simulink model "rccg_digitalTwin_scenario1"  (R2024a)
settings: Solver=VariableStepAuto  StartTime=0.0  StopTime=5  RelTol=1e-3
libraries: spsThreePhaseVIMeasurementLib x11, spsThreePhaseBreakerLib x9, spsThreePhaseDynamicLoadLib x7, spsSynchronousMachinepuStandardLib x2, spsThreePhaseParallelRLCLoadLib x2, spsThreePhaseTransformerTwoWindingsLib x1, spsExcitationSystemLib x1, spsHydraulicTurbineandGovernorLib x1, sps_lib x1
settings Model: Creator=dogba  LastModifiedBy=dogba

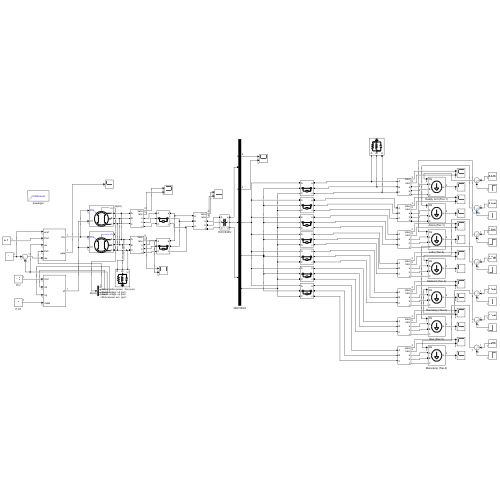
[thumbnail: Simulink's stored preview of the top-level diagram]
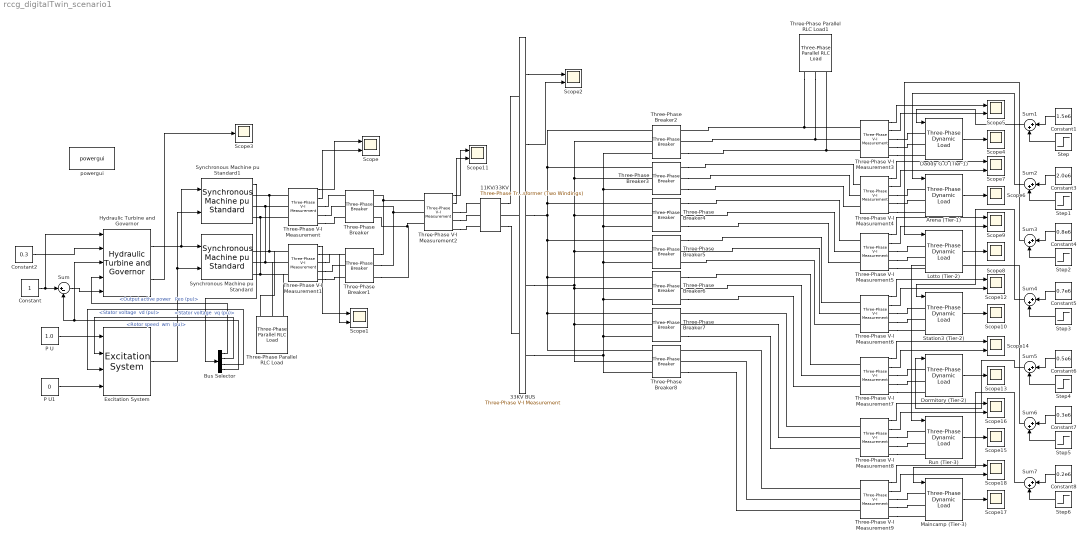
== system rccg_digitalTwin_scenario1 ==
  11KV/33KV : spsThreePhaseTransformerTwoWindingsLib/Three-Phase Transformer (Two Windings)  Winding1Connection=Yg  Winding2Connection=Yg  CoreType=Three single-phase transformers  SetSaturation=off  Hysteresis=off  DataFile='hysteresis'  SetInitialFlux=off  Measurements=None  UNITS=pu  NominalPower=[ 10e6 , 60 ]  Winding1=[ 11e3 , 0.002 , 0.08 ]  Winding2=[ 33e3 , 0.002 , 0.08 ]  Rm=500  Lm=500  L0=0.5  Saturation=[ 0,0 ; 0.0024,1.2 ; 1.0,1.52 ]  InitialFluxes=[ 0.8 , -0.8 , 0.7 ]  BreakLoop=off  DiscreteSolver=Trapezoidal iterative  DataType=off  TransfoNumber=1
  33KV BUS : spsThreePhaseVIMeasurementLib/Three-Phase V-I Measurement  VoltageMeasurement=phase-to-ground  SetLabelV=off  LabelV=Vabc  Vpu=off  VpuLL=off  CurrentMeasurement=yes  SetLabelI=off  LabelI=Iabc  Ipu=off  Pbase=100e6  Vbase=500e3  OutputType=Complex  PhasorSimulation=off  PSBequivalent=0
  Arena (Tier-1) : spsThreePhaseDynamicLoadLib/Three-Phase Dynamic Load  NominalVoltage=[ 415 50 ]  ActiveReactivePowers=[1.5e6 0.4e6]  PositiveSequence=[0.994 -11.8]  ExternalControl=on  NpNq=[1.3 2]  TimeConstants="[0  0  0  0]"  MinimumVoltage=0.7  Tfilter=1e-4  LoadFlowParameters=[4,0,0,0,0]
      settings: LibrarySourceBlock=|
      | sps_lib/Passives/Three-Phase
      | Dynamic Load
  Bus Selector : BusSelector  OutputSignals="Output active power   Peo (pu),dq0 components.Stator voltage  vd (pu),dq0 components.Stator voltage  vq (pu),Mechanical.Rotor speed  wm  (pu)"
  Constant : Constant
  Constant1 : Constant  Value=1.5e6
  Constant2 : Constant  Value=0.3
  Constant3 : Constant  Value=2.0e6
  Constant4 : Constant  Value=0.8e6
  Constant5 : Constant  Value=0.7e6
  Constant6 : Constant  Value=0.5e6
  Constant7 : Constant  Value=0.3e6
  Constant8 : Constant  Value=0.2e6
  Daddy G.O (Tier-1) : spsThreePhaseDynamicLoadLib/Three-Phase Dynamic Load  NominalVoltage=[ 415 50 ]  ActiveReactivePowers=[1.5e6 0.4e6]  PositiveSequence=[0.994 -11.8]  ExternalControl=on  NpNq=[1.3 2]  TimeConstants="[0  0  0  0]"  MinimumVoltage=0.7  Tfilter=1e-4  LoadFlowParameters=[4,0,0,0,0]
      settings: LibrarySourceBlock=|
      | sps_lib/Passives/Three-Phase
      | Dynamic Load
  Dormitory (Tier-2) : spsThreePhaseDynamicLoadLib/Three-Phase Dynamic Load  NominalVoltage=[ 415 50 ]  ActiveReactivePowers=[1.5e6 0.4e6]  PositiveSequence=[0.994 -11.8]  ExternalControl=on  NpNq=[1.3 2]  TimeConstants="[0  0  0  0]"  MinimumVoltage=0.7  Tfilter=1e-4  LoadFlowParameters=[4,0,0,0,0]
      settings: LibrarySourceBlock=|
      | sps_lib/Passives/Three-Phase
      | Dynamic Load
  Excitation System : spsExcitationSystemLib/Excitation System  tr=20e-3  reg=[ 300, 0.001 ]  exc=[ 1, 0 ]  tgr=[ 0, 0 ]  damp=[ 0.001, 0.1 ]  sat=[ 0, 0 ]  lim=[ -11.5, 11.5, 0 ]  v0="[1.0  1.28]"
      settings: LibrarySourceBlock=sps_lib/Electrical Machines/Synchronous Machine Control/Excitation System
  Hydraulic Turbine and Governor : spsHydraulicTurbineandGovernorLib/Hydraulic Turbine and Governor  sm="[ 10/3  0.07 ]"  gate="[  0.01  0.97518  -0.1  0.1 ]"  reg="[  0.05  1.163  0.105  0  0.01  ]"  hyd="[  0  2.67  ]"  dref=0  po=0.7516
      settings: LibrarySourceBlock=|
      | sps_lib/Electrical Machines/Synchronous Machine Control/Hydraulic Turbine
      | and Governor
  Lotto (Tier-2) : spsThreePhaseDynamicLoadLib/Three-Phase Dynamic Load  NominalVoltage=[ 415 50 ]  ActiveReactivePowers=[1.5e6 0.4e6]  PositiveSequence=[0.994 -11.8]  ExternalControl=on  NpNq=[1.3 2]  TimeConstants="[0  0  0  0]"  MinimumVoltage=0.7  Tfilter=1e-4  LoadFlowParameters=[4,0,0,0,0]
      settings: LibrarySourceBlock=|
      | sps_lib/Passives/Three-Phase
      | Dynamic Load
  Maincamp (Tier-3) : spsThreePhaseDynamicLoadLib/Three-Phase Dynamic Load  NominalVoltage=[ 415 50 ]  ActiveReactivePowers=[1.5e6 0.4e6]  PositiveSequence=[0.994 -11.8]  ExternalControl=on  NpNq=[1.3 2]  TimeConstants="[0  0  0  0]"  MinimumVoltage=0.7  Tfilter=1e-4  LoadFlowParameters=[4,0,0,0,0]
      settings: LibrarySourceBlock=|
      | sps_lib/Passives/Three-Phase
      | Dynamic Load
  P U : Constant  Value=1.0
  P U1 : Constant  Value=0
  Run (Tier-3) : spsThreePhaseDynamicLoadLib/Three-Phase Dynamic Load  NominalVoltage=[ 415 50 ]  ActiveReactivePowers=[1.5e6 0.4e6]  PositiveSequence=[0.994 -11.8]  ExternalControl=on  NpNq=[1.3 2]  TimeConstants="[0  0  0  0]"  MinimumVoltage=0.7  Tfilter=1e-4  LoadFlowParameters=[4,0,0,0,0]
      settings: LibrarySourceBlock=|
      | sps_lib/Passives/Three-Phase
      | Dynamic Load
  Scope{,1..2,5,7,9,11..12,14,16,18} (11 alike) : Scope  NumInputPorts=2
  Scope{3..4,6,8,10,13,15,17} (8 alike) : Scope
  "Station3 (Tier-2) " : spsThreePhaseDynamicLoadLib/Three-Phase Dynamic Load  NominalVoltage=[ 415 50 ]  ActiveReactivePowers=[1.5e6 0.4e6]  PositiveSequence=[0.994 -11.8]  ExternalControl=on  NpNq=[1.3 2]  TimeConstants="[0  0  0  0]"  MinimumVoltage=0.7  Tfilter=1e-4  LoadFlowParameters=[4,0,0,0,0]
      settings: LibrarySourceBlock=|
      | sps_lib/Passives/Three-Phase
      | Dynamic Load
  Step : Step  Time=2.5  After=0.78e6  SampleTime=0
  Step1 : Step  Time=2.5  After=1.6e6  SampleTime=0
  Step{2..6} (5 alike) : Step  Time=2.5  After=0  SampleTime=0
  Sum : Sum  Inputs=|+-
  Sum{1..7} (7 alike) : Sum  Inputs=|++
  Synchronous Machine pu Standard : spsSynchronousMachinepuStandardLib/Synchronous Machine pu Standard  PresetModel=No  MechanicalLoad=Mechanical power Pm  ShowDetailedParameters=on  RotorType=Salient-pole  Units=per unit standard parameters  MeasurementBus=off  NominalParameters=[5e6 11e3 50]  Reactances1=[ 1.81, 0.3, 0.23, 1.76, 0.65, 0.25, 0.15 ]  Reactances2=[2.24 0.17 0.12 1.02 0.13 0.08]  dAxisTimeConstants=Short-circuit  qAxisTimeConstants=Short-circuit  TimeConstants1="[ 4.4849  0.0681  0.1  ]"  TimeConstants2=[ 8.0, 0.03, 1.0, 0.07 ]  TimeConstants3="[  4.49  0.0681  0.0513  ]"  TimeConstants4=[ 8.0, 0.03, 0.3371, 0.0295 ]  TimeConstants5=[ 1.01, 0.053, 0.1 ]  TimeConstants6=[ 1.3201, 0.023, 1.0, 0.07 ]  TimeConstants7=[0.012 0.003 0.003]  TimeConstants8=[ 1.3201, 0.0231, 0.3371, 0.0295 ]  StatorResistance=0.037875  Mechanical=[0.1028 0.02056 2]  PolePairs=20  InitialConditions="[ 0  0  0  0  0  0  0  0  1 ]"  SetSaturation=on  Saturation=[0.6404,0.7127,0.8441,0.9214,0.9956,1.082,1.19,1.316,1.457;0.7,0.7698,0.8872,0.9466,0.9969,1.046,1.1,1.151,1.201]  LoadFlowParameters=[1,0,0,0,0]  TsPowergui=0  TsBlock=-1  IterativeModel=Trapezoidal non iterative  IterativeDiscreteModel=Trapezoidal non iterative  BusType=PV  Pref=0  Qref=0  Qmin=-inf  Qmax=inf  PLF=0  QLF=0
  Synchronous Machine pu Standard1 : spsSynchronousMachinepuStandardLib/Synchronous Machine pu Standard  PresetModel=No  MechanicalLoad=Mechanical power Pm  ShowDetailedParameters=on  RotorType=Salient-pole  Units=per unit standard parameters  MeasurementBus=off  NominalParameters=[5e6 11e3 50]  Reactances1=[ 1.81, 0.3, 0.23, 1.76, 0.65, 0.25, 0.15 ]  Reactances2=[2.24 0.17 0.12 1.02 0.13 0.08]  dAxisTimeConstants=Short-circuit  qAxisTimeConstants=Short-circuit  TimeConstants1="[ 4.4849  0.0681  0.1  ]"  TimeConstants2=[ 8.0, 0.03, 1.0, 0.07 ]  TimeConstants3="[  4.49  0.0681  0.0513  ]"  TimeConstants4=[ 8.0, 0.03, 0.3371, 0.0295 ]  TimeConstants5=[ 1.01, 0.053, 0.1 ]  TimeConstants6=[ 1.3201, 0.023, 1.0, 0.07 ]  TimeConstants7=[0.012 0.003 0.003]  TimeConstants8=[ 1.3201, 0.0231, 0.3371, 0.0295 ]  StatorResistance=0.037875  Mechanical=[0.1028 0.02056 2]  PolePairs=20  InitialConditions="[ 0  0  0  0  0  0  0  0  1 ]"  SetSaturation=on  Saturation=[0.6404,0.7127,0.8441,0.9214,0.9956,1.082,1.19,1.316,1.457;0.7,0.7698,0.8872,0.9466,0.9969,1.046,1.1,1.151,1.201]  LoadFlowParameters=[1,0,0,0,0]  TsPowergui=0  TsBlock=-1  IterativeModel=Trapezoidal non iterative  IterativeDiscreteModel=Trapezoidal non iterative  BusType=PV  Pref=0  Qref=0  Qmin=-inf  Qmax=inf  PLF=0  QLF=0
  Three-Phase Parallel RLC Load : spsThreePhaseParallelRLCLoadLib/Three-Phase Parallel RLC Load  LConnTagsString=A|B|C  Configuration=Y (grounded)  NominalVoltage=1000  Vabc=[1e3 1e3 1e3]  Vabcp=[1e3 1e3 1e3]  NominalFrequency=60  UnbalancedPower=off  ActivePower=10e3  InductivePower=100  CapacitivePower=100  Pabc=[10e3 9e3 11e3]  QLabc=[100 90 110]  QCabc=[100 90 110]  Pabcp=[10e3 9e3 11e3]  QLabcp=[100 90 110]  QCabcp=[100 90 110]  Measurements=None  LoadType=constant Z
  Three-Phase Parallel RLC Load1 : spsThreePhaseParallelRLCLoadLib/Three-Phase Parallel RLC Load  LConnTagsString=A|B|C  Configuration=Y (grounded)  NominalVoltage=1000  Vabc=[1e3 1e3 1e3]  Vabcp=[1e3 1e3 1e3]  NominalFrequency=60  UnbalancedPower=off  ActivePower=10e3  InductivePower=100  CapacitivePower=100  Pabc=[10e3 9e3 11e3]  QLabc=[100 90 110]  QCabc=[100 90 110]  Pabcp=[10e3 9e3 11e3]  QLabcp=[100 90 110]  QCabcp=[100 90 110]  Measurements=None  LoadType=constant Z
  Three-Phase V-I Measurement{,1..9} (10 alike) : spsThreePhaseVIMeasurementLib/Three-Phase V-I Measurement  VoltageMeasurement=phase-to-ground  SetLabelV=off  LabelV=Vabc  Vpu=off  VpuLL=off  CurrentMeasurement=yes  SetLabelI=off  LabelI=Iabc  Ipu=off  Pbase=100e6  Vbase=500e3  OutputType=Complex  PhasorSimulation=off  PSBequivalent=0
  Three-Phase Breaker{,1..8} (9 alike) : spsThreePhaseBreakerLib/Three-Phase Breaker  InitialState=closed  SwitchA=on  SwitchB=on  SwitchC=on  SwitchTimes="[1/60  5/60]"  External=off  BreakerResistance=0.01  SnubberResistance=1e6  SnubberCapacitance=inf  Measurements=None
  powergui : sps_lib/powergui  Priority=1  SimulationMode=Continuous  SampleTime=50e-6  frequency=60  Iterations=50  frequencyindice=50  Pbase=100e6  ErrMax=1e-4  UnitsV=kV  UnitsW=MW  buscounter=0  FunctionMessages=off  echomessages=off  EnableUseOfTLC=off  CurrentSourceSwitches=off  DisableSnubberDevices=off  DisableRonSwitches=off  DisableVfSwitches=off  DisplayEquations=off  AutomaticDiscreteSolvers=off  SolverType=Tustin/Backward Euler (TBE)  Interpol=off  ExternalGateDelay=off  methode=off  Ts=100  x0status=blocks  SPID=on  SwTol=0  HookPort=off  NonlinearTolerance=1e-4  nMaxIteration=100  ContinueOnMaxIteration=off  RestoreLinks=warning  ResistiveCurrentMeasurement=off  Frange=[0:2:500]  Ylog=off  Xlog=on  ShowGrid=off  save=off  variable=ZData  structure=0  ZoomFFT=off  StartTime=0.0  cycles=1  DisplayStyle=1  fundamental=60  FreqAxis=off  MaxFrequency=1000  frequencyindicesteady=1  RmsSteady=1  display=off
  wires:
  Excitation System/1 -> Synchronous Machine pu Standard1/2, Synchronous Machine pu Standard/2
  Hydraulic Turbine and Governor/1 -> Synchronous Machine pu Standard1/1, Synchronous Machine pu Standard/1
  P U/1 -> Excitation System/1
  P U1/1 -> Excitation System/4
  Three-Phase V-I Measurement/1 -> Scope/1
  Three-Phase V-I Measurement/2 -> Scope/2
  Three-Phase V-I Measurement1/1 -> Scope1/1
  Three-Phase V-I Measurement1/2 -> Scope1/2
  Synchronous Machine pu Standard1/1 -> Bus Selector/1
  Bus Selector/1 -> Hydraulic Turbine and Governor/4  "<Output active power   Peo (pu)>"
  Bus Selector/2 -> Excitation System/2  "<Stator voltage  vd (pu)>"
  Bus Selector/3 -> Excitation System/3  "<Stator voltage  vq (pu)>"
  Bus Selector/4 -> Sum/2, Hydraulic Turbine and Governor/3  "<Rotor speed  wm  (pu)>"
  Constant/1 -> Hydraulic Turbine and Governor/1, Sum/1
  Sum/1 -> Hydraulic Turbine and Governor/5
  Constant2/1 -> Hydraulic Turbine and Governor/2
  33KV BUS/1 -> Scope2/1
  33KV BUS/2 -> Scope2/2
  Hydraulic Turbine and Governor/2 -> Scope3/1
  Three-Phase V-I Measurement2/1 -> Scope11/1
  Three-Phase V-I Measurement2/2 -> Scope11/2
  Daddy G.O (Tier-1)/1 -> Scope4/1
  Three-Phase V-I Measurement3/1 -> Scope5/1
  Three-Phase V-I Measurement3/2 -> Scope5/2
  Three-Phase V-I Measurement4/2 -> Scope7/2
  Three-Phase V-I Measurement4/1 -> Scope7/1
  Arena (Tier-1)/1 -> Scope6/1
  Lotto (Tier-2)/1 -> Scope8/1
  Three-Phase V-I Measurement5/1 -> Scope9/1
  Three-Phase V-I Measurement5/2 -> Scope9/2
  Three-Phase V-I Measurement6/2 -> Scope12/2
  Three-Phase V-I Measurement6/1 -> Scope12/1
  "Station3 (Tier-2) "/1 -> Scope10/1
  Dormitory (Tier-2)/1 -> Scope13/1
  Three-Phase V-I Measurement7/1 -> Scope14/1
  Three-Phase V-I Measurement7/2 -> Scope14/2
  Three-Phase V-I Measurement8/2 -> Scope16/2
  Three-Phase V-I Measurement8/1 -> Scope16/1
  Run (Tier-3)/1 -> Scope15/1
  Maincamp (Tier-3)/1 -> Scope17/1
  Three-Phase V-I Measurement9/1 -> Scope18/1
  Three-Phase V-I Measurement9/2 -> Scope18/2
  Constant1/1 -> Sum1/1
  Step/1 -> Sum1/2
  Sum1/1 -> Daddy G.O (Tier-1)/1
  Sum2/1 -> Arena (Tier-1)/1
  Step1/1 -> Sum2/2
  Constant3/1 -> Sum2/1
  Constant5/1 -> Sum4/1
  Step3/1 -> Sum4/2
  Sum4/1 -> "Station3 (Tier-2) "/1
  Sum3/1 -> Lotto (Tier-2)/1
  Step2/1 -> Sum3/2
  Constant4/1 -> Sum3/1
  Constant7/1 -> Sum6/1
  Step5/1 -> Sum6/2
  Sum6/1 -> Run (Tier-3)/1
  Sum7/1 -> Maincamp (Tier-3)/1
  Step6/1 -> Sum7/2
  Constant8/1 -> Sum7/1
  Constant6/1 -> Sum5/1
  Step4/1 -> Sum5/2
  Sum5/1 -> Dormitory (Tier-2)/1
  connections:
  Three-Phase Breaker1/RConn1 -- Three-Phase Breaker/RConn1 -- Three-Phase V-I Measurement2/LConn1
  Three-Phase Breaker1/RConn2 -- Three-Phase Breaker/RConn2 -- Three-Phase V-I Measurement2/LConn2
  Three-Phase Breaker1/RConn3 -- Three-Phase V-I Measurement2/LConn3 -- Three-Phase Breaker/RConn3
  33KV BUS/LConn2 -- 11KV/33KV/RConn2
  11KV/33KV/RConn1 -- 33KV BUS/LConn1
  11KV/33KV/RConn3 -- 33KV BUS/LConn3
  Three-Phase V-I Measurement/LConn1 -- Three-Phase Parallel RLC Load/LConn1 -- Three-Phase V-I Measurement1/LConn1 -- Synchronous Machine pu Standard/RConn1 -- Synchronous Machine pu Standard1/RConn1
  Three-Phase V-I Measurement/LConn2 -- Synchronous Machine pu Standard1/RConn2 -- Three-Phase Parallel RLC Load/LConn2 -- Three-Phase V-I Measurement1/LConn2 -- Synchronous Machine pu Standard/RConn2
  Three-Phase V-I Measurement/LConn3 -- Three-Phase Parallel RLC Load/LConn3 -- Three-Phase V-I Measurement1/LConn3 -- Synchronous Machine pu Standard/RConn3 -- Synchronous Machine pu Standard1/RConn3
  Three-Phase V-I Measurement1/RConn2 -- Three-Phase Breaker1/LConn2
  Three-Phase V-I Measurement1/RConn3 -- Three-Phase Breaker1/LConn3
  Three-Phase V-I Measurement1/RConn1 -- Three-Phase Breaker1/LConn1
  Three-Phase V-I Measurement/RConn3 -- Three-Phase Breaker/LConn3
  Three-Phase V-I Measurement/RConn2 -- Three-Phase Breaker/LConn2
  Three-Phase V-I Measurement/RConn1 -- Three-Phase Breaker/LConn1
  Three-Phase Breaker8/LConn1 -- Three-Phase Breaker7/LConn1 -- Three-Phase Breaker6/LConn1 -- Three-Phase Breaker5/LConn1 -- 33KV BUS/RConn1 -- Three-Phase Breaker4/LConn1 -- Three-Phase Breaker3/LConn1 -- Three-Phase Breaker2/LConn1
  Three-Phase Breaker2/LConn2 -- Three-Phase Breaker3/LConn2 -- Three-Phase Breaker4/LConn2 -- Three-Phase Breaker5/LConn2 -- 33KV BUS/RConn2 -- Three-Phase Breaker6/LConn2 -- Three-Phase Breaker7/LConn2 -- Three-Phase Breaker8/LConn2
  Three-Phase Breaker2/LConn3 -- Three-Phase Breaker3/LConn3 -- Three-Phase Breaker8/LConn3 -- 33KV BUS/RConn3 -- Three-Phase Breaker7/LConn3 -- Three-Phase Breaker6/LConn3 -- Three-Phase Breaker5/LConn3 -- Three-Phase Breaker4/LConn3
  Three-Phase V-I Measurement2/RConn1 -- 11KV/33KV/LConn1
  Three-Phase V-I Measurement2/RConn2 -- 11KV/33KV/LConn2
  Three-Phase V-I Measurement2/RConn3 -- 11KV/33KV/LConn3
  Three-Phase Parallel RLC Load1/LConn1 -- Three-Phase Breaker2/RConn1 -- Three-Phase V-I Measurement3/LConn1
  Three-Phase Parallel RLC Load1/LConn2 -- Three-Phase V-I Measurement3/LConn2 -- Three-Phase Breaker2/RConn2
  Three-Phase Breaker2/RConn3 -- Three-Phase Parallel RLC Load1/LConn3 -- Three-Phase V-I Measurement3/LConn3
  Three-Phase V-I Measurement3/RConn3 -- Daddy G.O (Tier-1)/LConn3
  Three-Phase V-I Measurement3/RConn2 -- Daddy G.O (Tier-1)/LConn2
  Three-Phase V-I Measurement3/RConn1 -- Daddy G.O (Tier-1)/LConn1
  Three-Phase V-I Measurement4/RConn1 -- Arena (Tier-1)/LConn1
  Three-Phase V-I Measurement4/RConn3 -- Arena (Tier-1)/LConn3
  Three-Phase V-I Measurement4/RConn2 -- Arena (Tier-1)/LConn2
  Three-Phase V-I Measurement5/RConn2 -- Lotto (Tier-2)/LConn2
  Three-Phase V-I Measurement5/RConn3 -- Lotto (Tier-2)/LConn3
  Three-Phase V-I Measurement5/RConn1 -- Lotto (Tier-2)/LConn1
  Three-Phase V-I Measurement6/RConn1 -- "Station3 (Tier-2) "/LConn1
  Three-Phase V-I Measurement6/RConn3 -- "Station3 (Tier-2) "/LConn3
  Three-Phase V-I Measurement6/RConn2 -- "Station3 (Tier-2) "/LConn2
  Three-Phase V-I Measurement7/RConn2 -- Dormitory (Tier-2)/LConn2
  Three-Phase V-I Measurement7/RConn3 -- Dormitory (Tier-2)/LConn3
  Three-Phase V-I Measurement7/RConn1 -- Dormitory (Tier-2)/LConn1
  Three-Phase V-I Measurement8/RConn3 -- Run (Tier-3)/LConn3
  Three-Phase V-I Measurement8/RConn2 -- Run (Tier-3)/LConn2
  Three-Phase V-I Measurement8/RConn1 -- Run (Tier-3)/LConn1
  Three-Phase V-I Measurement9/RConn1 -- Maincamp (Tier-3)/LConn1
  Three-Phase V-I Measurement9/RConn2 -- Maincamp (Tier-3)/LConn2
  Three-Phase V-I Measurement9/RConn3 -- Maincamp (Tier-3)/LConn3
  Three-Phase Breaker3/RConn1 -- Three-Phase V-I Measurement4/LConn1
  Three-Phase Breaker3/RConn2 -- Three-Phase V-I Measurement4/LConn2
  Three-Phase Breaker3/RConn3 -- Three-Phase V-I Measurement4/LConn3
  Three-Phase Breaker4/RConn1 -- Three-Phase V-I Measurement5/LConn1
  Three-Phase Breaker4/RConn2 -- Three-Phase V-I Measurement5/LConn2
  Three-Phase Breaker4/RConn3 -- Three-Phase V-I Measurement5/LConn3
  Three-Phase Breaker5/RConn1 -- Three-Phase V-I Measurement6/LConn1
  Three-Phase Breaker5/RConn2 -- Three-Phase V-I Measurement6/LConn2
  Three-Phase V-I Measurement6/LConn3 -- Three-Phase Breaker5/RConn3
  Three-Phase Breaker6/RConn1 -- Three-Phase V-I Measurement7/LConn1
  Three-Phase Breaker6/RConn2 -- Three-Phase V-I Measurement7/LConn2
  Three-Phase Breaker6/RConn3 -- Three-Phase V-I Measurement7/LConn3
  Three-Phase V-I Measurement8/LConn1 -- Three-Phase Breaker7/RConn1
  Three-Phase Breaker7/RConn2 -- Three-Phase V-I Measurement8/LConn2
  Three-Phase Breaker7/RConn3 -- Three-Phase V-I Measurement8/LConn3
  Three-Phase V-I Measurement9/LConn1 -- Three-Phase Breaker8/RConn1
  Three-Phase V-I Measurement9/LConn2 -- Three-Phase Breaker8/RConn2
  Three-Phase Breaker8/RConn3 -- Three-Phase V-I Measurement9/LConn3
